simulink model "motorsimRight"  (R2024b)
settings: Solver=VariableStepAuto  StartTime=0.0  StopTime=3  RelTol=1e-3
model workspace (MAT data in the model file):
  K = Simulink.Parameter
  K.Value = 4.2
  K.Complexity = 'real'
  K.Dimensions = [1 1]
  K.DataType = 'auto'
values from neighbouring files (symbols this model uses):
  K = 4.12    [runControlSimRight.m]    (also in runmotorsim.m = 2.2; runmotorsim2.m; runmotorsimRight.m)
  sigma = 14    [runControlSimRight.m]    (also in runmotorsim.m = 5; runmotorsim2.m; runmotorsimRight.m)
settings Model: Creator=bensmithva  LastModifiedBy=bensmithva

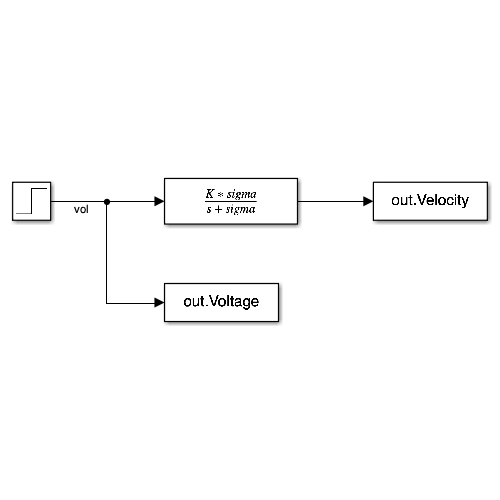
[thumbnail: Simulink's stored preview of the top-level diagram]
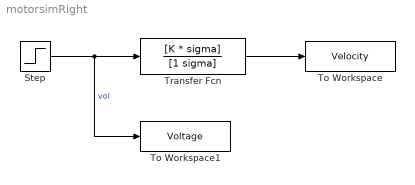
== system motorsimRight ==
  Step : Step  SampleTime=0
  To Workspace : ToWorkspace  VariableName=Velocity  SaveFormat=Timeseries  SampleTime=-1
  To Workspace1 : ToWorkspace  VariableName=Voltage  SaveFormat=Timeseries  SampleTime=-1
  Transfer Fcn : TransferFcn  Numerator=[K * sigma]  Denominator=[1 sigma]
  wires:
  Step/1 -> Transfer Fcn/1, To Workspace1/1  "vol"
  Transfer Fcn/1 -> To Workspace/1
